simulink model "Test"  (Simulink 7.2)
settings: Solver=FixedStepDiscrete  StartTime=0.0  StopTime=10  RelTol=1e-6  AbsTol=1e-6
InitFcn:
  | clear('all');
libraries: simulink x1
settings Model: Creator=Andreas Schellenberg  LastModifiedBy=Andreas
settings DataIOCC: LimitDataPoints=off  SaveFormat=StructureWithTime  SaveState=on  SignalLogging=off  SignalLoggingName=sigsOut  OutputOption=SpecifiedOutputTimes  OutputTimes=t
settings OptimizationCC: InitFltsAndDblsToZero=on
settings DebuggingCC: SaveWithParameterizedLinksMsg=none  SignalResolutionControl=TryResolveAllWithWarning  SolverPrmCheckMsg=none  MultiTaskDSMMsg=warning  MultiTaskCondExecSysMsg=none  StrictBusMsg=None
settings HardwareCC: TargetUnknown=on
settings RTWCC: IncludeERTFirstTime=on

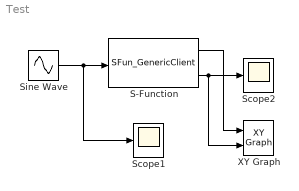
== system Test ==
  S-Function : S-Function  FunctionName=SFun_GenericClient  Parameters=ipAddr,ipPort,dataSize  EnableBusSupport=off  mask(GenericClient Element){ipAddr='127.0.0.1', ipPort=8090, dataSize=256}
      mask prompts: ipAddr "IP Address of Server"; ipPort "IP Port Number of Server"; dataSize "Size of Data Arrays"
      mask Display: disp('GenericClient\nElement');
  Scope1 : Scope
      settings: TimeRange=10  YMin=-2.5  YMax=2.5
  Scope2 : Scope
      settings: TimeRange=10  YMin=-1.5  YMax=2
  Sine Wave : Sin  Amplitude=2  Frequency=pi  SampleTime=0.01
  XY Graph : simulink/Sinks/XY Graph  SystemSampleTime=-1  xmin=-2.5  xmax=2.5  ymin=-2  ymax=2  st=-1
  wires:
  Sine Wave/1 -> S-Function/1, Scope1/1
  S-Function/2 -> Scope2/1, XY Graph/2
  S-Function/1 -> XY Graph/1
